simulink model "AR4_robotv5"  (R2021a)
settings: Solver=VariableStepAuto  StartTime=0.0  StopTime=13.7896  RelTol=1e-3
undefined symbols (not defined in the file or in its folder): B, Levenberg, Marquardt, sigbuilder_block, Spline, X, Y, Z
libraries: sm_lib x612, nesl_utility x123, robotcorelib x28, simulink_extras x19, simulink x17, robotmaniplib x9
(part 13 of 14)

== system AR4_robotv5/Subsystem8/link4 ==
  Inertia : sm_lib/Body Elements/Inertia  InertiaType=Custom  Mass=0.330915774998875  MassUnits=kg  CenterOfMass=[0, 0, 0]  CenterOfMassUnits=m  MomentsOfInertia=[0.0007707144648363029, 0.000143595801102121, 0.00078144566914053]  MomentsOfInertiaUnits=kg*m^2  ProductsOfInertia=[6.92144604392256e-05, -9.03681380466358e-09, -5.83780279549621e-08]  ProductsOfInertiaUnits=kg*m^2  GraphicType=None  MarkerShape=Inertia  MarkerSize=20  GraphicVisPropType=SimpleVisualProperties  GraphicDiffuseColor=[0.5 0.5 0.5]  GraphicSpecularColor=[0.5 0.5 0.5 1.0]  GraphicAmbientColor=[0.15 0.15 0.15 1.0]  GraphicEmissiveColor=[0.0 0.0 0.0 1.0]  GraphicShininess=75  GraphicOpacity=1.0
  InertiaOriginTransform : sm_lib/Frames and Transforms/Rigid Transform  TranslationMethod=Cartesian  TranslationStandardOffset=0  TranslationLengthUnit=m  TranslationStandardAxis=+Z  TranslationCartesianOffset=[1.65972746341003e-06, 0.114308868744708, -0.00196391551724488]  TranslationROffset=0  TranslationROffsetUnits=m  TranslationZOffset=0  TranslationZOffsetUnits=m  TranslationThetaOffset=0  TranslationThetaOffsetUnits=deg  RotationMethod=RotationSequence  RotationAngleUnits=deg  RotationStandardAxis=+Z  RotationAngle=0.0  RotationArbitraryAxis=[0 0 1]  FollAlignAxisA=+X  BaseAlignAxisA=+Y  FollAlignAxisB=+Y  BaseAlignAxisB=+Z  RotationSequenceAxes=BaseAxes  RotationSequence=XYZ  RotationSequenceAngles=[0, 0, 0]  RotationSequenceAnglesUnits=rad  RotationMatrix=[1 0 0; 0 1 0; 0 0 1]
  ReferenceFrame : sm_lib/Frames and Transforms/Reference Frame
  Visual : sm_lib/Body Elements/File Solid  ExtGeomFileName=AR4_robotv5/meshes/link4.STL  UnitType=Custom  ExtGeomFileUnits=m  StepReaderType=HEX  ExportConvexHullGeometry=off  InertiaType=Custom  Mass=0  MassUnits=kg  CenterOfMass=[0, 0, 0]  CenterOfMassUnits=m  MomentsOfInertia=[0, 0, 0]  MomentsOfInertiaUnits=kg*m^2  ProductsOfInertia=[0, 0, 0]  ProductsOfInertiaUnits=kg*m^2  BasedOnType=DensityFromFile  Density=1000  DensityUnits=kg/m^3  DoExposeReferenceFrame=on  SerializedFrames=<Frames/>  GraphicType=FromGeometry  MarkerShape=Sphere  MarkerSize=10  GraphicVisPropType=SimpleVisualProperties  GraphicDiffuseColor=[0.792156862745098, 0.819607843137255, 0.933333333333333]  GraphicSpecularColor=[0.5 0.5 0.5 1.0]  GraphicAmbientColor=[0.15 0.15 0.15 1.0]  GraphicEmissiveColor=[0.0 0.0 0.0 1.0]  GraphicShininess=75  GraphicOpacity=1
  VisualOriginTransform : sm_lib/Frames and Transforms/Rigid Transform  TranslationMethod=Cartesian  TranslationStandardOffset=0  TranslationLengthUnit=m  TranslationStandardAxis=+Z  TranslationCartesianOffset=[0, 0, 0]  TranslationROffset=0  TranslationROffsetUnits=m  TranslationZOffset=0  TranslationZOffsetUnits=m  TranslationThetaOffset=0  TranslationThetaOffsetUnits=deg  RotationMethod=RotationSequence  RotationAngleUnits=deg  RotationStandardAxis=+Z  RotationAngle=0.0  RotationArbitraryAxis=[0 0 1]  FollAlignAxisA=+X  BaseAlignAxisA=+Y  FollAlignAxisB=+Y  BaseAlignAxisB=+Z  RotationSequenceAxes=BaseAxes  RotationSequence=XYZ  RotationSequenceAngles=[0, 0, 0]  RotationSequenceAnglesUnits=rad  RotationMatrix=[1 0 0; 0 1 0; 0 0 1]
  j4_AxisInvTransform : sm_lib/Frames and Transforms/Rigid Transform  TranslationMethod=Cartesian  TranslationStandardOffset=0  TranslationLengthUnit=m  TranslationStandardAxis=+Z  TranslationCartesianOffset=[0, 0, 0]  TranslationROffset=0  TranslationROffsetUnits=m  TranslationZOffset=0  TranslationZOffsetUnits=m  TranslationThetaOffset=0  TranslationThetaOffsetUnits=deg  RotationMethod=ArbitraryAxis  RotationAngleUnits=rad  RotationStandardAxis=+Z  RotationAngle=1.570796326794897  RotationArbitraryAxis=[-1, 0, 0]  FollAlignAxisA=+X  BaseAlignAxisA=+Y  FollAlignAxisB=+Y  BaseAlignAxisB=+Z  RotationSequenceAxes=FollowerAxes  RotationSequence=XYX  RotationSequenceAngles=[0 0 0]  RotationSequenceAnglesUnits=deg  RotationMatrix=[1 0 0; 0 1 0; 0 0 1]
  j5_AxisTransform : sm_lib/Frames and Transforms/Rigid Transform  TranslationMethod=Cartesian  TranslationStandardOffset=0  TranslationLengthUnit=m  TranslationStandardAxis=+Z  TranslationCartesianOffset=[0, 0, 0]  TranslationROffset=0  TranslationROffsetUnits=m  TranslationZOffset=0  TranslationZOffsetUnits=m  TranslationThetaOffset=0  TranslationThetaOffsetUnits=deg  RotationMethod=ArbitraryAxis  RotationAngleUnits=rad  RotationStandardAxis=+Z  RotationAngle=1.570796326794897  RotationArbitraryAxis=[-1, 0, 0]  FollAlignAxisA=+X  BaseAlignAxisA=+Y  FollAlignAxisB=+Y  BaseAlignAxisB=+Z  RotationSequenceAxes=FollowerAxes  RotationSequence=XYX  RotationSequenceAngles=[0 0 0]  RotationSequenceAnglesUnits=deg  RotationMatrix=[1 0 0; 0 1 0; 0 0 1]
  j5_OriginTransform : sm_lib/Frames and Transforms/Rigid Transform  TranslationMethod=Cartesian  TranslationStandardOffset=0  TranslationLengthUnit=m  TranslationStandardAxis=+Z  TranslationCartesianOffset=[0, 0.225041312909753, 0.0007499997333115]  TranslationROffset=0  TranslationROffsetUnits=m  TranslationZOffset=0  TranslationZOffsetUnits=m  TranslationThetaOffset=0  TranslationThetaOffsetUnits=deg  RotationMethod=RotationSequence  RotationAngleUnits=deg  RotationStandardAxis=+Z  RotationAngle=0.0  RotationArbitraryAxis=[0 0 1]  FollAlignAxisA=+X  BaseAlignAxisA=+Y  FollAlignAxisB=+Y  BaseAlignAxisB=+Z  RotationSequenceAxes=BaseAxes  RotationSequence=XYZ  RotationSequenceAngles=[1.57079631189374, -0.000843332253807779, 0]  RotationSequenceAnglesUnits=rad  RotationMatrix=[1 0 0; 0 1 0; 0 0 1]
  F : PMIOPort  Side=Left
  F1 : PMIOPort  Port=2  Side=Right
  connections:
  j5_AxisTransform/LConn1 -- j5_OriginTransform/RConn1
  j5_AxisTransform/RConn1 -- F1/RConn1
  j4_AxisInvTransform/RConn1 -- F/RConn1
  Visual/RConn1 -- VisualOriginTransform/RConn1
  j5_OriginTransform/LConn1 -- j4_AxisInvTransform/LConn1 -- VisualOriginTransform/LConn1 -- ReferenceFrame/RConn1 -- InertiaOriginTransform/LConn1
  Inertia/RConn1 -- InertiaOriginTransform/RConn1

== system AR4_robotv5/Subsystem8/link5 ==
  Inertia : sm_lib/Body Elements/Inertia  InertiaType=Custom  Mass=0.0245034490928621  MassUnits=kg  CenterOfMass=[0, 0, 0]  CenterOfMassUnits=m  MomentsOfInertia=[9.036336684299629e-06, 5.7526255063883e-06, 1.2157538793257e-05]  MomentsOfInertiaUnits=kg*m^2  ProductsOfInertia=[-2.03350961333318e-08, -2.14953206266449e-09, 9.04257798543254e-09]  ProductsOfInertiaUnits=kg*m^2  GraphicType=None  MarkerShape=Inertia  MarkerSize=20  GraphicVisPropType=SimpleVisualProperties  GraphicDiffuseColor=[0.5 0.5 0.5]  GraphicSpecularColor=[0.5 0.5 0.5 1.0]  GraphicAmbientColor=[0.15 0.15 0.15 1.0]  GraphicEmissiveColor=[0.0 0.0 0.0 1.0]  GraphicShininess=75  GraphicOpacity=1.0
  InertiaOriginTransform : sm_lib/Frames and Transforms/Rigid Transform  TranslationMethod=Cartesian  TranslationStandardOffset=0  TranslationLengthUnit=m  TranslationStandardAxis=+Z  TranslationCartesianOffset=[4.46631409203313e-05, 0.0010582355958296, -0.000637441503684444]  TranslationROffset=0  TranslationROffsetUnits=m  TranslationZOffset=0  TranslationZOffsetUnits=m  TranslationThetaOffset=0  TranslationThetaOffsetUnits=deg  RotationMethod=RotationSequence  RotationAngleUnits=deg  RotationStandardAxis=+Z  RotationAngle=0.0  RotationArbitraryAxis=[0 0 1]  FollAlignAxisA=+X  BaseAlignAxisA=+Y  FollAlignAxisB=+Y  BaseAlignAxisB=+Z  RotationSequenceAxes=BaseAxes  RotationSequence=XYZ  RotationSequenceAngles=[0, 0, 0]  RotationSequenceAnglesUnits=rad  RotationMatrix=[1 0 0; 0 1 0; 0 0 1]
  ReferenceFrame : sm_lib/Frames and Transforms/Reference Frame
  Visual : sm_lib/Body Elements/File Solid  ExtGeomFileName=AR4_robotv5/meshes/link5.STL  UnitType=Custom  ExtGeomFileUnits=m  StepReaderType=HEX  ExportConvexHullGeometry=off  InertiaType=Custom  Mass=0  MassUnits=kg  CenterOfMass=[0, 0, 0]  CenterOfMassUnits=m  MomentsOfInertia=[0, 0, 0]  MomentsOfInertiaUnits=kg*m^2  ProductsOfInertia=[0, 0, 0]  ProductsOfInertiaUnits=kg*m^2  BasedOnType=DensityFromFile  Density=1000  DensityUnits=kg/m^3  DoExposeReferenceFrame=on  SerializedFrames=<Frames/>  GraphicType=FromGeometry  MarkerShape=Sphere  MarkerSize=10  GraphicVisPropType=SimpleVisualProperties  GraphicDiffuseColor=[0.792156862745098, 0.819607843137255, 0.933333333333333]  GraphicSpecularColor=[0.5 0.5 0.5 1.0]  GraphicAmbientColor=[0.15 0.15 0.15 1.0]  GraphicEmissiveColor=[0.0 0.0 0.0 1.0]  GraphicShininess=75  GraphicOpacity=1
  VisualOriginTransform : sm_lib/Frames and Transforms/Rigid Transform  TranslationMethod=Cartesian  TranslationStandardOffset=0  TranslationLengthUnit=m  TranslationStandardAxis=+Z  TranslationCartesianOffset=[0, 0, 0]  TranslationROffset=0  TranslationROffsetUnits=m  TranslationZOffset=0  TranslationZOffsetUnits=m  TranslationThetaOffset=0  TranslationThetaOffsetUnits=deg  RotationMethod=RotationSequence  RotationAngleUnits=deg  RotationStandardAxis=+Z  RotationAngle=0.0  RotationArbitraryAxis=[0 0 1]  FollAlignAxisA=+X  BaseAlignAxisA=+Y  FollAlignAxisB=+Y  BaseAlignAxisB=+Z  RotationSequenceAxes=BaseAxes  RotationSequence=XYZ  RotationSequenceAngles=[0, 0, 0]  RotationSequenceAnglesUnits=rad  RotationMatrix=[1 0 0; 0 1 0; 0 0 1]
  j5_AxisInvTransform : sm_lib/Frames and Transforms/Rigid Transform  TranslationMethod=Cartesian  TranslationStandardOffset=0  TranslationLengthUnit=m  TranslationStandardAxis=+Z  TranslationCartesianOffset=[0, 0, 0]  TranslationROffset=0  TranslationROffsetUnits=m  TranslationZOffset=0  TranslationZOffsetUnits=m  TranslationThetaOffset=0  TranslationThetaOffsetUnits=deg  RotationMethod=ArbitraryAxis  RotationAngleUnits=rad  RotationStandardAxis=+Z  RotationAngle=1.570796326794897  RotationArbitraryAxis=[-1, 0, 0]  FollAlignAxisA=+X  BaseAlignAxisA=+Y  FollAlignAxisB=+Y  BaseAlignAxisB=+Z  RotationSequenceAxes=FollowerAxes  RotationSequence=XYX  RotationSequenceAngles=[0 0 0]  RotationSequenceAnglesUnits=deg  RotationMatrix=[1 0 0; 0 1 0; 0 0 1]
  j6_AxisTransform : sm_lib/Frames and Transforms/Rigid Transform  TranslationMethod=Cartesian  TranslationStandardOffset=0  TranslationLengthUnit=m  TranslationStandardAxis=+Z  TranslationCartesianOffset=[0, 0, 0]  TranslationROffset=0  TranslationROffsetUnits=m  TranslationZOffset=0  TranslationZOffsetUnits=m  TranslationThetaOffset=0  TranslationThetaOffsetUnits=deg  RotationMethod=ArbitraryAxis  RotationAngleUnits=rad  RotationStandardAxis=+Z  RotationAngle=0  RotationArbitraryAxis=[1, 0, 0]  FollAlignAxisA=+X  BaseAlignAxisA=+Y  FollAlignAxisB=+Y  BaseAlignAxisB=+Z  RotationSequenceAxes=FollowerAxes  RotationSequence=XYX  RotationSequenceAngles=[0 0 0]  RotationSequenceAnglesUnits=deg  RotationMatrix=[1 0 0; 0 1 0; 0 0 1]
  j6_OriginTransform : sm_lib/Frames and Transforms/Rigid Transform  TranslationMethod=Cartesian  TranslationStandardOffset=0  TranslationLengthUnit=m  TranslationStandardAxis=+Z  TranslationCartesianOffset=[0, 0, 0]  TranslationROffset=0  TranslationROffsetUnits=m  TranslationZOffset=0  TranslationZOffsetUnits=m  TranslationThetaOffset=0  TranslationThetaOffsetUnits=deg  RotationMethod=RotationSequence  RotationAngleUnits=deg  RotationStandardAxis=+Z  RotationAngle=0.0  RotationArbitraryAxis=[0 0 1]  FollAlignAxisA=+X  BaseAlignAxisA=+Y  FollAlignAxisB=+Y  BaseAlignAxisB=+Z  RotationSequenceAxes=BaseAxes  RotationSequence=XYZ  RotationSequenceAngles=[0, 0, 3.14159265358979]  RotationSequenceAnglesUnits=rad  RotationMatrix=[1 0 0; 0 1 0; 0 0 1]
  F : PMIOPort  Side=Left
  F1 : PMIOPort  Port=2  Side=Right
  connections:
  j6_AxisTransform/LConn1 -- j6_OriginTransform/RConn1
  j6_AxisTransform/RConn1 -- F1/RConn1
  j5_AxisInvTransform/RConn1 -- F/RConn1
  Visual/RConn1 -- VisualOriginTransform/RConn1
  j6_OriginTransform/LConn1 -- j5_AxisInvTransform/LConn1 -- VisualOriginTransform/LConn1 -- ReferenceFrame/RConn1 -- InertiaOriginTransform/LConn1
  Inertia/RConn1 -- InertiaOriginTransform/RConn1

== system AR4_robotv5/Subsystem8/link6 ==
  Inertia : sm_lib/Body Elements/Inertia  InertiaType=Custom  Mass=0.121376042767568  MassUnits=kg  CenterOfMass=[0, 0, 0]  CenterOfMassUnits=m  MomentsOfInertia=[3.53039178237827e-05, 1.81330403322111e-05, 4.26315107565952e-05]  MomentsOfInertiaUnits=kg*m^2  ProductsOfInertia=[-2.21518225549172e-07, -4.47726039625278e-07, -4.7308746638171e-08]  ProductsOfInertiaUnits=kg*m^2  GraphicType=None  MarkerShape=Inertia  MarkerSize=20  GraphicVisPropType=SimpleVisualProperties  GraphicDiffuseColor=[0.5 0.5 0.5]  GraphicSpecularColor=[0.5 0.5 0.5 1.0]  GraphicAmbientColor=[0.15 0.15 0.15 1.0]  GraphicEmissiveColor=[0.0 0.0 0.0 1.0]  GraphicShininess=75  GraphicOpacity=1.0
  InertiaOriginTransform : sm_lib/Frames and Transforms/Rigid Transform  TranslationMethod=Cartesian  TranslationStandardOffset=0  TranslationLengthUnit=m  TranslationStandardAxis=+Z  TranslationCartesianOffset=[-0.00160633858276565, -0.000457062617008543, -0.0587695487539506]  TranslationROffset=0  TranslationROffsetUnits=m  TranslationZOffset=0  TranslationZOffsetUnits=m  TranslationThetaOffset=0  TranslationThetaOffsetUnits=deg  RotationMethod=RotationSequence  RotationAngleUnits=deg  RotationStandardAxis=+Z  RotationAngle=0.0  RotationArbitraryAxis=[0 0 1]  FollAlignAxisA=+X  BaseAlignAxisA=+Y  FollAlignAxisB=+Y  BaseAlignAxisB=+Z  RotationSequenceAxes=BaseAxes  RotationSequence=XYZ  RotationSequenceAngles=[0, 0, 0]  RotationSequenceAnglesUnits=rad  RotationMatrix=[1 0 0; 0 1 0; 0 0 1]
  ReferenceFrame : sm_lib/Frames and Transforms/Reference Frame
  Visual : sm_lib/Body Elements/File Solid  ExtGeomFileName=AR4_robotv5/meshes/link6.STL  UnitType=Custom  ExtGeomFileUnits=m  StepReaderType=HEX  ExportConvexHullGeometry=off  InertiaType=Custom  Mass=0  MassUnits=kg  CenterOfMass=[0, 0, 0]  CenterOfMassUnits=m  MomentsOfInertia=[0, 0, 0]  MomentsOfInertiaUnits=kg*m^2  ProductsOfInertia=[0, 0, 0]  ProductsOfInertiaUnits=kg*m^2  BasedOnType=DensityFromFile  Density=1000  DensityUnits=kg/m^3  DoExposeReferenceFrame=on  SerializedFrames=<Frames/>  GraphicType=FromGeometry  MarkerShape=Sphere  MarkerSize=10  GraphicVisPropType=SimpleVisualProperties  GraphicDiffuseColor=[0.792156862745098, 0.819607843137255, 0.933333333333333]  GraphicSpecularColor=[0.5 0.5 0.5 1.0]  GraphicAmbientColor=[0.15 0.15 0.15 1.0]  GraphicEmissiveColor=[0.0 0.0 0.0 1.0]  GraphicShininess=75  GraphicOpacity=1
  VisualOriginTransform : sm_lib/Frames and Transforms/Rigid Transform  TranslationMethod=Cartesian  TranslationStandardOffset=0  TranslationLengthUnit=m  TranslationStandardAxis=+Z  TranslationCartesianOffset=[0, 0, 0]  TranslationROffset=0  TranslationROffsetUnits=m  TranslationZOffset=0  TranslationZOffsetUnits=m  TranslationThetaOffset=0  TranslationThetaOffsetUnits=deg  RotationMethod=RotationSequence  RotationAngleUnits=deg  RotationStandardAxis=+Z  RotationAngle=0.0  RotationArbitraryAxis=[0 0 1]  FollAlignAxisA=+X  BaseAlignAxisA=+Y  FollAlignAxisB=+Y  BaseAlignAxisB=+Z  RotationSequenceAxes=BaseAxes  RotationSequence=XYZ  RotationSequenceAngles=[0, 0, 0]  RotationSequenceAnglesUnits=rad  RotationMatrix=[1 0 0; 0 1 0; 0 0 1]
  j6_AxisInvTransform : sm_lib/Frames and Transforms/Rigid Transform  TranslationMethod=Cartesian  TranslationStandardOffset=0  TranslationLengthUnit=m  TranslationStandardAxis=+Z  TranslationCartesianOffset=[0, 0, 0]  TranslationROffset=0  TranslationROffsetUnits=m  TranslationZOffset=0  TranslationZOffsetUnits=m  TranslationThetaOffset=0  TranslationThetaOffsetUnits=deg  RotationMethod=ArbitraryAxis  RotationAngleUnits=rad  RotationStandardAxis=+Z  RotationAngle=0  RotationArbitraryAxis=[1, 0, 0]  FollAlignAxisA=+X  BaseAlignAxisA=+Y  FollAlignAxisB=+Y  BaseAlignAxisB=+Z  RotationSequenceAxes=FollowerAxes  RotationSequence=XYX  RotationSequenceAngles=[0 0 0]  RotationSequenceAnglesUnits=deg  RotationMatrix=[1 0 0; 0 1 0; 0 0 1]
  j7_OriginTransform : sm_lib/Frames and Transforms/Rigid Transform  TranslationMethod=Cartesian  TranslationStandardOffset=0  TranslationLengthUnit=m  TranslationStandardAxis=+Z  TranslationCartesianOffset=[0, -0.000201201957805657, -0.0848321039170631]  TranslationROffset=0  TranslationROffsetUnits=m  TranslationZOffset=0  TranslationZOffsetUnits=m  TranslationThetaOffset=0  TranslationThetaOffsetUnits=deg  RotationMethod=RotationSequence  RotationAngleUnits=deg  RotationStandardAxis=+Z  RotationAngle=0.0  RotationArbitraryAxis=[0 0 1]  FollAlignAxisA=+X  BaseAlignAxisA=+Y  FollAlignAxisB=+Y  BaseAlignAxisB=+Z  RotationSequenceAxes=BaseAxes  RotationSequence=XYZ  RotationSequenceAngles=[0, 1.5707963267949, 0]  RotationSequenceAnglesUnits=rad  RotationMatrix=[1 0 0; 0 1 0; 0 0 1]
  F : PMIOPort  Side=Left
  F1 : PMIOPort  Port=2  Side=Right
  connections:
  j7_OriginTransform/RConn1 -- F1/RConn1
  j6_AxisInvTransform/RConn1 -- F/RConn1
  Visual/RConn1 -- VisualOriginTransform/RConn1
  j7_OriginTransform/LConn1 -- j6_AxisInvTransform/LConn1 -- VisualOriginTransform/LConn1 -- ReferenceFrame/RConn1 -- InertiaOriginTransform/LConn1
  Inertia/RConn1 -- InertiaOriginTransform/RConn1

== system AR4_robotv5/Subsystem8/link7 ==
  Inertia : sm_lib/Body Elements/Inertia  InertiaType=Custom  Mass=4.28541445828409e-05  MassUnits=kg  CenterOfMass=[0, 0, 0]  CenterOfMassUnits=m  MomentsOfInertia=[3.26374304335892e-11, 3.40574299802589e-10, 3.40574299802589e-10]  MomentsOfInertiaUnits=kg*m^2  ProductsOfInertia=[2.22599419002211e-28, 4.70953291237086e-24, 1.38439272082023e-24]  ProductsOfInertiaUnits=kg*m^2  GraphicType=None  MarkerShape=Inertia  MarkerSize=20  GraphicVisPropType=SimpleVisualProperties  GraphicDiffuseColor=[0.5 0.5 0.5]  GraphicSpecularColor=[0.5 0.5 0.5 1.0]  GraphicAmbientColor=[0.15 0.15 0.15 1.0]  GraphicEmissiveColor=[0.0 0.0 0.0 1.0]  GraphicShininess=75  GraphicOpacity=1.0
  InertiaOriginTransform : sm_lib/Frames and Transforms/Rigid Transform  TranslationMethod=Cartesian  TranslationStandardOffset=0  TranslationLengthUnit=m  TranslationStandardAxis=+Z  TranslationCartesianOffset=[0.00401715386268953, -1.82145964977565e-17, -1.11022302462516e-16]  TranslationROffset=0  TranslationROffsetUnits=m  TranslationZOffset=0  TranslationZOffsetUnits=m  TranslationThetaOffset=0  TranslationThetaOffsetUnits=deg  RotationMethod=RotationSequence  RotationAngleUnits=deg  RotationStandardAxis=+Z  RotationAngle=0.0  RotationArbitraryAxis=[0 0 1]  FollAlignAxisA=+X  BaseAlignAxisA=+Y  FollAlignAxisB=+Y  BaseAlignAxisB=+Z  RotationSequenceAxes=BaseAxes  RotationSequence=XYZ  RotationSequenceAngles=[0, 0, 0]  RotationSequenceAnglesUnits=rad  RotationMatrix=[1 0 0; 0 1 0; 0 0 1]
  ReferenceFrame : sm_lib/Frames and Transforms/Reference Frame
  Visual : sm_lib/Body Elements/File Solid  ExtGeomFileName=AR4_robotv5/meshes/link7.STL  UnitType=Custom  ExtGeomFileUnits=m  StepReaderType=HEX  ExportConvexHullGeometry=off  InertiaType=Custom  Mass=0  MassUnits=kg  CenterOfMass=[0, 0, 0]  CenterOfMassUnits=m  MomentsOfInertia=[0, 0, 0]  MomentsOfInertiaUnits=kg*m^2  ProductsOfInertia=[0, 0, 0]  ProductsOfInertiaUnits=kg*m^2  BasedOnType=DensityFromFile  Density=1000  DensityUnits=kg/m^3  DoExposeReferenceFrame=on  SerializedFrames=<Frames/>  GraphicType=FromGeometry  MarkerShape=Sphere  MarkerSize=10  GraphicVisPropType=SimpleVisualProperties  GraphicDiffuseColor=[0.792156862745098, 0.819607843137255, 0.933333333333333]  GraphicSpecularColor=[0.5 0.5 0.5 1.0]  GraphicAmbientColor=[0.15 0.15 0.15 1.0]  GraphicEmissiveColor=[0.0 0.0 0.0 1.0]  GraphicShininess=75  GraphicOpacity=1
  VisualOriginTransform : sm_lib/Frames and Transforms/Rigid Transform  TranslationMethod=Cartesian  TranslationStandardOffset=0  TranslationLengthUnit=m  TranslationStandardAxis=+Z  TranslationCartesianOffset=[0, 0, 0]  TranslationROffset=0  TranslationROffsetUnits=m  TranslationZOffset=0  TranslationZOffsetUnits=m  TranslationThetaOffset=0  TranslationThetaOffsetUnits=deg  RotationMethod=RotationSequence  RotationAngleUnits=deg  RotationStandardAxis=+Z  RotationAngle=0.0  RotationArbitraryAxis=[0 0 1]  FollAlignAxisA=+X  BaseAlignAxisA=+Y  FollAlignAxisB=+Y  BaseAlignAxisB=+Z  RotationSequenceAxes=BaseAxes  RotationSequence=XYZ  RotationSequenceAngles=[0, 0, 0]  RotationSequenceAnglesUnits=rad  RotationMatrix=[1 0 0; 0 1 0; 0 0 1]
  F : PMIOPort  Side=Left
  connections:
  Visual/RConn1 -- VisualOriginTransform/RConn1
  F/RConn1 -- VisualOriginTransform/LConn1 -- ReferenceFrame/RConn1 -- InertiaOriginTransform/LConn1
  Inertia/RConn1 -- InertiaOriginTransform/RConn1

== matlab function AR4_robotv5/Subsystem6/MATLAB Function4 ==
  data: theta1 input; H output; theta2 input; theta3 input; theta4 input; theta5 input; theta6 input; X output; Y output; Z output; Rz output; Ry output; Rx output
function [H, X, Y, Z, Rz, Ry, Rx] = forward_kinematics_AR4(theta1, theta2, theta3, theta4, theta5, theta6)
% forward_kinematics_AR4 Computes the forward kinematics for the AR4 robot.
%
%   [H, X, Y, Z, Rz, Ry, Rx] = forward_kinematics_AR4(theta1, theta2, theta3, theta4, theta5, theta6)
%
%   Inputs:
%       theta1, theta2, theta3, theta4, theta5, theta6 - Joint angles (degrees)
%
%   Outputs:
%       H  - 4x4 homogeneous transformation matrix of the end-effector (mm)
%       X, Y, Z - End-effector position coordinates (mm)
%       Rz, Ry, Rx - End-effector orientation angles in degrees (ZYX Euler angles)
%
%   The AR4 robot parameters (in mm) used here are:
%       a1 = 64.2;   a2 = 305;    a3 = 0;
%       d1 = 151.27; d4 = 225.04; d6 = 37.9;
%
%   The DH parameters are defined as:
%       Joint 1: [theta1,         d1, a1, -90]
%       Joint 2: [theta2 - 90,     0,  a2,   0]
%       Joint 3: [theta3 + 180,    0,  a3,  90]
%       Joint 4: [theta4,         d4,  0,   -90]
%       Joint 5: [theta5,          0,  0,    90]
%       Joint 6: [theta6,         d6,  0,     0]

    %% Robot parameters
    a1 = 64.2;     a2 = 305;    a3 = 0;
    d1 = 151.27;   d4 = 225.04; d6 = 84.832;

    %% DH parameters
    DH1 = [theta1,       d1, a1, -90];
    DH2 = [theta2 - 90,  0,  a2,   0];
    DH3 = [theta3 + 180, 0,  a3,  90];
    DH4 = [theta4,       d4,  0,   -90];
    DH5 = [theta5,        0,  0,    90];
    DH6 = [theta6,       d6,  0,     0];

    %% Compute transformations
    A1 = computeDH(DH1);
    A2 = computeDH(DH2);
    A3 = computeDH(DH3);
    A4 = computeDH(DH4);
    A5 = computeDH(DH5);
    A6 = computeDH(DH6);

    H = A1 * A2 * A3 * A4 * A5 * A6;

    %% Extract position
    X = H(1,4);
    Y = H(2,4);
    Z = H(3,4);

    %% Extract orientation (ZYX Euler angles in degrees)
    R = H(1:3, 1:3);
    
    % Calculate Ry (pitch)
    Ry = atan2d(-R(3,1), sqrt(R(3,2)^2 + R(3,3)^2));
    
    % Check for gimbal lock (pitch near ±90°)
    if abs(abs(Ry) - 90) < eps
        % Gimbal lock case - set yaw to 0 and compute roll from alternate terms
        Rz = 0;
        Rx = atan2d(R(1,2), R(2,2));
    else
        % Normal case
        Rz = atan2d(R(2,1), R(1,1));
        Rx = atan2d(R(3,2), R(3,3));
    end
end

function A = computeDH(dh)
    theta = dh(1);
    d     = dh(2);
    a     = dh(3);
    alpha = dh(4);
    
    A = [cosd(theta), -sind(theta)*cosd(alpha),  sind(theta)*sind(alpha), a*cosd(theta);
         sind(theta),  cosd(theta)*cosd(alpha), -cosd(theta)*sind(alpha), a*sind(theta);
         0,            sind(alpha),             cosd(alpha),             d;
         0,            0,                       0,                       1];
end

== matlab function AR4_robotv5/MATLAB Function3 ==
  data: theta1 input; H output; theta2 input; theta3 input; theta4 input; theta5 input; theta6 input; X output; Y output; Z output; Rz output; Ry output; Rx output
function [H, X, Y, Z, Rz, Ry, Rx] = forward_kinematics_AR4(theta1, theta2, theta3, theta4, theta5, theta6)
% forward_kinematics_AR4 Computes the forward kinematics for the AR4 robot.
%
%   [H, X, Y, Z, Rz, Ry, Rx] = forward_kinematics_AR4(theta1, theta2, theta3, theta4, theta5, theta6)
%
%   Inputs:
%       theta1, theta2, theta3, theta4, theta5, theta6 - Joint angles (degrees)
%
%   Outputs:
%       H  - 4x4 homogeneous transformation matrix of the end-effector (mm)
%       X, Y, Z - End-effector position coordinates (mm)
%       Rz, Ry, Rx - End-effector orientation angles in degrees (ZYX Euler angles)
%
%   The AR4 robot parameters (in mm) used here are:
%       a1 = 64.2;   a2 = 305;    a3 = 0;
%       d1 = 151.27; d4 = 225.04; d6 = 37.9;
%
%   The DH parameters are defined as:
%       Joint 1: [theta1,         d1, a1, -90]
%       Joint 2: [theta2 - 90,     0,  a2,   0]
%       Joint 3: [theta3 + 180,    0,  a3,  90]
%       Joint 4: [theta4,         d4,  0,   -90]
%       Joint 5: [theta5,          0,  0,    90]
%       Joint 6: [theta6,         d6,  0,     0]

    %% Robot parameters
    a1 = 64.2;     a2 = 305;    a3 = 0;
    d1 = 151.27;   d4 = 225.04; d6 = 84.832;

    %% DH parameters
    DH1 = [theta1,       d1, a1, -90];
    DH2 = [theta2 - 90,  0,  a2,   0];
    DH3 = [theta3 + 180, 0,  a3,  90];
    DH4 = [theta4,       d4,  0,   -90];
    DH5 = [theta5,        0,  0,    90];
    DH6 = [theta6,       d6,  0,     0];

    %% Compute transformations
    A1 = computeDH(DH1);
    A2 = computeDH(DH2);
    A3 = computeDH(DH3);
    A4 = computeDH(DH4);
    A5 = computeDH(DH5);
    A6 = computeDH(DH6);

    H = A1 * A2 * A3 * A4 * A5 * A6;

    %% Extract position
    X = H(1,4);
    Y = H(2,4);
    Z = H(3,4);

    %% Extract orientation (ZYX Euler angles in degrees)
    R = H(1:3, 1:3);
    
    % Calculate Ry (pitch)
    Ry = atan2d(-R(3,1), sqrt(R(3,2)^2 + R(3,3)^2));
    
    % Check for gimbal lock (pitch near ±90°)
    if abs(abs(Ry) - 90) < eps
        % Gimbal lock case - set yaw to 0 and compute roll from alternate terms
        Rz = 0;
        Rx = atan2d(R(1,2), R(2,2));
    else
        % Normal case
        Rz = atan2d(R(2,1), R(1,1));
        Rx = atan2d(R(3,2), R(3,3));
    end
end

function A = computeDH(dh)
    theta = dh(1);
    d     = dh(2);
    a     = dh(3);
    alpha = dh(4);
    
    A = [cosd(theta), -sind(theta)*cosd(alpha),  sind(theta)*sind(alpha), a*cosd(theta);
         sind(theta),  cosd(theta)*cosd(alpha), -cosd(theta)*sind(alpha), a*sind(theta);
         0,            sind(alpha),             cosd(alpha),             d;
         0,            0,                       0,                       1];
end

== matlab function AR4_robotv5/MATLAB Function6 ==
  data: theta1 input; H output; theta2 input; theta3 input; theta4 input; theta5 input; theta6 input; X output; Y output; Z output; Rz output; Ry output; Rx output
function [H, X, Y, Z, Rz, Ry, Rx] = forward_kinematics_AR4(theta1, theta2, theta3, theta4, theta5, theta6)
% forward_kinematics_AR4 Computes the forward kinematics for the AR4 robot.
%
%   [H, X, Y, Z, Rz, Ry, Rx] = forward_kinematics_AR4(theta1, theta2, theta3, theta4, theta5, theta6)
%
%   Inputs:
%       theta1, theta2, theta3, theta4, theta5, theta6 - Joint angles (degrees)
%
%   Outputs:
%       H  - 4x4 homogeneous transformation matrix of the end-effector (mm)
%       X, Y, Z - End-effector position coordinates (mm)
%       Rz, Ry, Rx - End-effector orientation angles in degrees (ZYX Euler angles)
%
%   The AR4 robot parameters (in mm) used here are:
%       a1 = 64.2;   a2 = 305;    a3 = 0;
%       d1 = 151.27; d4 = 225.04; d6 = 37.9;
%
%   The DH parameters are defined as:
%       Joint 1: [theta1,         d1, a1, -90]
%       Joint 2: [theta2 - 90,     0,  a2,   0]
%       Joint 3: [theta3 + 180,    0,  a3,  90]
%       Joint 4: [theta4,         d4,  0,   -90]
%       Joint 5: [theta5,          0,  0,    90]
%       Joint 6: [theta6,         d6,  0,     0]

    %% Robot parameters
    a1 = 64.2;     a2 = 305;    a3 = 0;
    d1 = 151.27;   d4 = 225.04; d6 = 84.832;

    %% DH parameters
    DH1 = [theta1,       d1, a1, -90];
    DH2 = [theta2 - 90,  0,  a2,   0];
    DH3 = [theta3 + 180, 0,  a3,  90];
    DH4 = [theta4,       d4,  0,   -90];
    DH5 = [theta5,        0,  0,    90];
    DH6 = [theta6,       d6,  0,     0];

    %% Compute transformations
    A1 = computeDH(DH1);
    A2 = computeDH(DH2);
    A3 = computeDH(DH3);
    A4 = computeDH(DH4);
    A5 = computeDH(DH5);
    A6 = computeDH(DH6);

    H = A1 * A2 * A3 * A4 * A5 * A6;

    %% Extract position
    X = H(1,4);
    Y = H(2,4);
    Z = H(3,4);

    %% Extract orientation (ZYX Euler angles in degrees)
    R = H(1:3, 1:3);
    
    % Calculate Ry (pitch)
    Ry = atan2d(-R(3,1), sqrt(R(3,2)^2 + R(3,3)^2));
    
    % Check for gimbal lock (pitch near ±90°)
    if abs(abs(Ry) - 90) < eps
        % Gimbal lock case - set yaw to 0 and compute roll from alternate terms
        Rz = 0;
        Rx = atan2d(R(1,2), R(2,2));
    else
        % Normal case
        Rz = atan2d(R(2,1), R(1,1));
        Rx = atan2d(R(3,2), R(3,3));
    end
end

function A = computeDH(dh)
    theta = dh(1);
    d     = dh(2);
    a     = dh(3);
    alpha = dh(4);
    
    A = [cosd(theta), -sind(theta)*cosd(alpha),  sind(theta)*sind(alpha), a*cosd(theta);
         sind(theta),  cosd(theta)*cosd(alpha), -cosd(theta)*sind(alpha), a*sind(theta);
         0,            sind(alpha),             cosd(alpha),             d;
         0,            0,                       0,                       1];
end

== matlab function AR4_robotv5/Subsystem12/MATLAB Function4 ==
  data: theta1 input; H output; theta2 input; theta3 input; theta4 input; theta5 input; theta6 input; X output; Y output; Z output; Rz output; Ry output; Rx output
function [H, X, Y, Z, Rz, Ry, Rx] = forward_kinematics_AR4(theta1, theta2, theta3, theta4, theta5, theta6)
% forward_kinematics_AR4 Computes the forward kinematics for the AR4 robot.
%
%   [H, X, Y, Z, Rz, Ry, Rx] = forward_kinematics_AR4(theta1, theta2, theta3, theta4, theta5, theta6)
%
%   Inputs:
%       theta1, theta2, theta3, theta4, theta5, theta6 - Joint angles (degrees)
%
%   Outputs:
%       H  - 4x4 homogeneous transformation matrix of the end-effector (mm)
%       X, Y, Z - End-effector position coordinates (mm)
%       Rz, Ry, Rx - End-effector orientation angles in degrees (ZYX Euler angles)
%
%   The AR4 robot parameters (in mm) used here are:
%       a1 = 64.2;   a2 = 305;    a3 = 0;
%       d1 = 151.27; d4 = 225.04; d6 = 37.9;
%
%   The DH parameters are defined as:
%       Joint 1: [theta1,         d1, a1, -90]
%       Joint 2: [theta2 - 90,     0,  a2,   0]
%       Joint 3: [theta3 + 180,    0,  a3,  90]
%       Joint 4: [theta4,         d4,  0,   -90]
%       Joint 5: [theta5,          0,  0,    90]
%       Joint 6: [theta6,         d6,  0,     0]

    %% Robot parameters
    a1 = 64.2;     a2 = 305;    a3 = 0;
    d1 = 151.27;   d4 = 225.04; d6 = 84.832;

    %% DH parameters
    DH1 = [theta1,       d1, a1, -90];
    DH2 = [theta2 - 90,  0,  a2,   0];
    DH3 = [theta3 + 180, 0,  a3,  90];
    DH4 = [theta4,       d4,  0,   -90];
    DH5 = [theta5,        0,  0,    90];
    DH6 = [theta6,       d6,  0,     0];

    %% Compute transformations
    A1 = computeDH(DH1);
    A2 = computeDH(DH2);
    A3 = computeDH(DH3);
    A4 = computeDH(DH4);
    A5 = computeDH(DH5);
    A6 = computeDH(DH6);

    H = A1 * A2 * A3 * A4 * A5 * A6;

    %% Extract position
    X = H(1,4);
    Y = H(2,4);
    Z = H(3,4);

    %% Extract orientation (ZYX Euler angles in degrees)
    R = H(1:3, 1:3);
    
    % Calculate Ry (pitch)
    Ry = atan2d(-R(3,1), sqrt(R(3,2)^2 + R(3,3)^2));
    
    % Check for gimbal lock (pitch near ±90°)
    if abs(abs(Ry) - 90) < eps
        % Gimbal lock case - set yaw to 0 and compute roll from alternate terms
        Rz = 0;
        Rx = atan2d(R(1,2), R(2,2));
    else
        % Normal case
        Rz = atan2d(R(2,1), R(1,1));
        Rx = atan2d(R(3,2), R(3,3));
    end
end

function A = computeDH(dh)
    theta = dh(1);
    d     = dh(2);
    a     = dh(3);
    alpha = dh(4);
    
    A = [cosd(theta), -sind(theta)*cosd(alpha),  sind(theta)*sind(alpha), a*cosd(theta);
         sind(theta),  cosd(theta)*cosd(alpha), -cosd(theta)*sind(alpha), a*sind(theta);
         0,            sind(alpha),             cosd(alpha),             d;
         0,            0,                       0,                       1];
end

== matlab function AR4_robotv5/MATLAB Function ==
  data: q input; stopFlag input
function store_joint_angles(q, stopFlag)
%#codegen

% Inputs:
%   q        : 6x1 joint angle vector
%   stopFlag : 1 if simulation is ending, 0 otherwise

persistent Q_table idx
coder.extrinsic('assignin')  % Let Simulink use this for simulation only

if isempty(Q_table)
    Q_table = zeros(10000, 6);  % Allocate storage
    idx = 1;
end

% Store current joint angles
if idx <= size(Q_table, 1)
    Q_table(idx, :) = q(:)';
    idx = idx + 1;
end

% At end of simulation, export to base workspace
if stopFlag
    assignin('base', 'JointAngleLog', Q_table(1:idx-1, :));
end

== matlab function AR4_robotv5/MATLAB Function4 ==
  data: q input; stopFlag input
function store_joint_angles(q, stopFlag)
%#codegen

% Inputs:
%   q        : 6x1 joint angle vector
%   stopFlag : 1 if simulation is ending, 0 otherwise

persistent Q_table idx
coder.extrinsic('assignin')  % Let Simulink use this for simulation only

if isempty(Q_table)
    Q_table = zeros(10000, 6);  % Allocate storage
    idx = 1;
end

% Store current joint angles
if idx <= size(Q_table, 1)
    Q_table(idx, :) = q(:)';
    idx = idx + 1;
end

% At end of simulation, export to base workspace
if stopFlag
    assignin('base', 'JointAngleLog', Q_table(1:idx-1, :));
end

== matlab function AR4_robotv5/MATLAB Function7 ==
  data: theta1 input; H output; theta2 input; theta3 input; theta4 input; theta5 input; theta6 input; q output; Rz output; Ry output; Rx output
function [H, q, Rz, Ry, Rx] = forward_kinematics_AR4(theta1, theta2, theta3, theta4, theta5, theta6)
% forward_kinematics_AR4 Computes the forward kinematics for the AR4 robot.
%
%   [H, X, Y, Z, Rz, Ry, Rx] = forward_kinematics_AR4(theta1, theta2, theta3, theta4, theta5, theta6)
%
%   Inputs:
%       theta1, theta2, theta3, theta4, theta5, theta6 - Joint angles (degrees)
%
%   Outputs:
%       H  - 4x4 homogeneous transformation matrix of the end-effector (mm)
%       X, Y, Z - End-effector position coordinates (mm)
%       Rz, Ry, Rx - End-effector orientation angles in degrees (ZYX Euler angles)
%
%   The AR4 robot parameters (in mm) used here are:
%       a1 = 64.2;   a2 = 305;    a3 = 0;
%       d1 = 151.27; d4 = 225.04; d6 = 37.9;
%
%   The DH parameters are defined as:
%       Joint 1: [theta1,         d1, a1, -90]
%       Joint 2: [theta2 - 90,     0,  a2,   0]
%       Joint 3: [theta3 + 180,    0,  a3,  90]
%       Joint 4: [theta4,         d4,  0,   -90]
%       Joint 5: [theta5,          0,  0,    90]
%       Joint 6: [theta6,         d6,  0,     0]

    %% Robot parameters
    a1 = 64.2;     a2 = 305;    a3 = 0;
    d1 = 151.27;   d4 = 225.04; d6 = 84.832;

    %% DH parameters
    DH1 = [theta1,       d1, a1, -90];
    DH2 = [theta2 - 90,  0,  a2,   0];
    DH3 = [theta3 + 180, 0,  a3,  90];
    DH4 = [theta4,       d4,  0,   -90];
    DH5 = [theta5,        0,  0,    90];
    DH6 = [theta6,       d6,  0,     0];

    %% Compute transformations
    A1 = computeDH(DH1);
    A2 = computeDH(DH2);
    A3 = computeDH(DH3);
    A4 = computeDH(DH4);
    A5 = computeDH(DH5);
    A6 = computeDH(DH6);

    H = A1 * A2 * A3 * A4 * A5 * A6;

    %% Extract position
   
        q = [H(1,4); H(2,4); H(3,4)];  % ← Cartesian position vector

    

    %% Extract orientation (ZYX Euler angles in degrees)
    R = H(1:3, 1:3);
    
    % Calculate Ry (pitch)
    Ry = atan2d(-R(3,1), sqrt(R(3,2)^2 + R(3,3)^2));
    
    % Check for gimbal lock (pitch near ±90°)
    if abs(abs(Ry) - 90) < eps
        % Gimbal lock case - set yaw to 0 and compute roll from alternate terms
        Rz = 0;
        Rx = atan2d(R(1,2), R(2,2));
    else
        % Normal case c
        Rz = atan2d(R(2,1), R(1,1));
        Rx = atan2d(R(3,2), R(3,3));
    end
end

function A = computeDH(dh)
    theta = dh(1);
    d     = dh(2);
    a     = dh(3);
    alpha = dh(4);
    
    A = [cosd(theta), -sind(theta)*cosd(alpha),  sind(theta)*sind(alpha), a*cosd(theta);
         sind(theta),  cosd(theta)*cosd(alpha), -cosd(theta)*sind(alpha), a*sind(theta);
         0,            sind(alpha),             cosd(alpha),             d;
         0,            0,                       0,                       1];
end

== matlab function AR4_robotv5/MATLAB Function8 ==
  data: theta1 input; H output; theta2 input; theta3 input; theta4 input; theta5 input; theta6 input; q output; Rz output; Ry output; Rx output
function [H, q, Rz, Ry, Rx] = forward_kinematics_AR4(theta1, theta2, theta3, theta4, theta5, theta6)
% forward_kinematics_AR4 Computes the forward kinematics for the AR4 robot.
%
%   [H, X, Y, Z, Rz, Ry, Rx] = forward_kinematics_AR4(theta1, theta2, theta3, theta4, theta5, theta6)
%
%   Inputs:
%       theta1, theta2, theta3, theta4, theta5, theta6 - Joint angles (degrees)
%
%   Outputs:
%       H  - 4x4 homogeneous transformation matrix of the end-effector (mm)
%       X, Y, Z - End-effector position coordinates (mm)
%       Rz, Ry, Rx - End-effector orientation angles in degrees (ZYX Euler angles)
%
%   The AR4 robot parameters (in mm) used here are:
%       a1 = 64.2;   a2 = 305;    a3 = 0;
%       d1 = 151.27; d4 = 225.04; d6 = 37.9;
%
%   The DH parameters are defined as:
%       Joint 1: [theta1,         d1, a1, -90]
%       Joint 2: [theta2 - 90,     0,  a2,   0]
%       Joint 3: [theta3 + 180,    0,  a3,  90]
%       Joint 4: [theta4,         d4,  0,   -90]
%       Joint 5: [theta5,          0,  0,    90]
%       Joint 6: [theta6,         d6,  0,     0]

    %% Robot parameters
    a1 = 64.2;     a2 = 305;    a3 = 0;
    d1 = 151.27;   d4 = 225.04; d6 = 84.832;

    %% DH parameters
    DH1 = [theta1,       d1, a1, -90];
    DH2 = [theta2 - 90,  0,  a2,   0];
    DH3 = [theta3 + 180, 0,  a3,  90];
    DH4 = [theta4,       d4,  0,   -90];
    DH5 = [theta5,        0,  0,    90];
    DH6 = [theta6,       d6,  0,     0];

    %% Compute transformations
    A1 = computeDH(DH1);
    A2 = computeDH(DH2);
    A3 = computeDH(DH3);
    A4 = computeDH(DH4);
    A5 = computeDH(DH5);
    A6 = computeDH(DH6);

    H = A1 * A2 * A3 * A4 * A5 * A6;

    %% Extract position
   
        q = [H(1,4); H(2,4); H(3,4)];  % ← Cartesian position vector

    

    %% Extract orientation (ZYX Euler angles in degrees)
    R = H(1:3, 1:3);
    
    % Calculate Ry (pitch)
    Ry = atan2d(-R(3,1), sqrt(R(3,2)^2 + R(3,3)^2));
    
    % Check for gimbal lock (pitch near ±90°)
    if abs(abs(Ry) - 90) < eps
        % Gimbal lock case - set yaw to 0 and compute roll from alternate terms
        Rz = 0;
        Rx = atan2d(R(1,2), R(2,2));
    else
        % Normal case c
        Rz = atan2d(R(2,1), R(1,1));
        Rx = atan2d(R(3,2), R(3,3));
    end
end

function A = computeDH(dh)
    theta = dh(1);
    d     = dh(2);
    a     = dh(3);
    alpha = dh(4);
    
    A = [cosd(theta), -sind(theta)*cosd(alpha),  sind(theta)*sind(alpha), a*cosd(theta);
         sind(theta),  cosd(theta)*cosd(alpha), -cosd(theta)*sind(alpha), a*sind(theta);
         0,            sind(alpha),             cosd(alpha),             d;
         0,            0,                       0,                       1];
end

== matlab function AR4_robotv5/MATLAB Function9 ==
  data: theta1 input; H output; theta2 input; theta3 input; theta4 input; theta5 input; theta6 input; q output; Rz output; Ry output; Rx output
function [H, q, Rz, Ry, Rx] = forward_kinematics_AR4(theta1, theta2, theta3, theta4, theta5, theta6)
% forward_kinematics_AR4 Computes the forward kinematics for the AR4 robot.
%
%   [H, X, Y, Z, Rz, Ry, Rx] = forward_kinematics_AR4(theta1, theta2, theta3, theta4, theta5, theta6)
%
%   Inputs:
%       theta1, theta2, theta3, theta4, theta5, theta6 - Joint angles (degrees)
%
%   Outputs:
%       H  - 4x4 homogeneous transformation matrix of the end-effector (mm)
%       X, Y, Z - End-effector position coordinates (mm)
%       Rz, Ry, Rx - End-effector orientation angles in degrees (ZYX Euler angles)
%
%   The AR4 robot parameters (in mm) used here are:
%       a1 = 64.2;   a2 = 305;    a3 = 0;
%       d1 = 151.27; d4 = 225.04; d6 = 37.9;
%
%   The DH parameters are defined as:
%       Joint 1: [theta1,         d1, a1, -90]
%       Joint 2: [theta2 - 90,     0,  a2,   0]
%       Joint 3: [theta3 + 180,    0,  a3,  90]
%       Joint 4: [theta4,         d4,  0,   -90]
%       Joint 5: [theta5,          0,  0,    90]
%       Joint 6: [theta6,         d6,  0,     0]

    %% Robot parameters
    a1 = 64.2;     a2 = 305;    a3 = 0;
    d1 = 151.27;   d4 = 225.04; d6 = 84.832;

    %% DH parameters
    DH1 = [theta1,       d1, a1, -90];
    DH2 = [theta2 ,  0,  a2,   0];
    DH3 = [theta3 , 0,  a3,  90];
    DH4 = [theta4,       d4,  0,   -90];
    DH5 = [theta5,        0,  0,    90];
    DH6 = [theta6,       d6,  0,     0];

    %% Compute transformations
    A1 = computeDH(DH1);
    A2 = computeDH(DH2);
    A3 = computeDH(DH3);
    A4 = computeDH(DH4);
    A5 = computeDH(DH5);
    A6 = computeDH(DH6);

    H = A1 * A2 * A3 * A4 * A5 * A6;

    %% Extract position
   
        q = [H(1,4); H(2,4); H(3,4)];  % ← Cartesian position vector

    

    %% Extract orientation (ZYX Euler angles in degrees)
    R = H(1:3, 1:3);
    
    % Calculate Ry (pitch)
    Ry = atan2d(-R(3,1), sqrt(R(3,2)^2 + R(3,3)^2));
    
    % Check for gimbal lock (pitch near ±90°)
    if abs(abs(Ry) - 90) < eps
        % Gimbal lock case - set yaw to 0 and compute roll from alternate terms
        Rz = 0;
        Rx = atan2d(R(1,2), R(2,2));
    else
        % Normal case c
        Rz = atan2d(R(2,1), R(1,1));
        Rx = atan2d(R(3,2), R(3,3));
    end
end

function A = computeDH(dh)
    theta = dh(1);
    d     = dh(2);
    a     = dh(3);
    alpha = dh(4);
    
    A = [cosd(theta), -sind(theta)*cosd(alpha),  sind(theta)*sind(alpha), a*cosd(theta);
         sind(theta),  cosd(theta)*cosd(alpha), -cosd(theta)*sind(alpha), a*sind(theta);
         0,            sind(alpha),             cosd(alpha),             d;
         0,            0,                       0,                       1];
end

== matlab function AR4_robotv5/MATLAB Function10 ==
  data: theta1 input; H output; theta2 input; theta3 input; theta4 input; theta5 input; theta6 input; q output; Rz output; Ry output; Rx output
function [H, q, Rz, Ry, Rx] = forward_kinematics_AR4(theta1, theta2, theta3, theta4, theta5, theta6)
% forward_kinematics_AR4 Computes the forward kinematics for the AR4 robot.
%
%   [H, X, Y, Z, Rz, Ry, Rx] = forward_kinematics_AR4(theta1, theta2, theta3, theta4, theta5, theta6)
%
%   Inputs:
%       theta1, theta2, theta3, theta4, theta5, theta6 - Joint angles (degrees)
%
%   Outputs:
%       H  - 4x4 homogeneous transformation matrix of the end-effector (mm)
%       X, Y, Z - End-effector position coordinates (mm)
%       Rz, Ry, Rx - End-effector orientation angles in degrees (ZYX Euler angles)
%
%   The AR4 robot parameters (in mm) used here are:
%       a1 = 64.2;   a2 = 305;    a3 = 0;
%       d1 = 151.27; d4 = 225.04; d6 = 37.9;
%
%   The DH parameters are defined as:
%       Joint 1: [theta1,         d1, a1, -90]
%       Joint 2: [theta2 - 90,     0,  a2,   0]
%       Joint 3: [theta3 + 180,    0,  a3,  90]
%       Joint 4: [theta4,         d4,  0,   -90]
%       Joint 5: [theta5,          0,  0,    90]
%       Joint 6: [theta6,         d6,  0,     0]

    %% Robot parameters
    a1 = 64.2;     a2 = 305;    a3 = 0;
    d1 = 151.27;   d4 = 225.04; d6 = 84.832;

    %% DH parameters
    DH1 = [theta1,       d1, a1, -90];
    DH2 = [theta2 - 90,  0,  a2,   0];
    DH3 = [theta3 + 180, 0,  a3,  90];
    DH4 = [theta4,       d4,  0,   -90];
    DH5 = [theta5,        0,  0,    90];
    DH6 = [theta6,       d6,  0,     0];

    %% Compute transformations
    A1 = computeDH(DH1);
    A2 = computeDH(DH2);
    A3 = computeDH(DH3);
    A4 = computeDH(DH4);
    A5 = computeDH(DH5);
    A6 = computeDH(DH6);

    H = A1 * A2 * A3 * A4 * A5 * A6;

    %% Extract position
   
        q = [H(1,4); H(2,4); H(3,4)];  % ← Cartesian position vector

    

    %% Extract orientation (ZYX Euler angles in degrees)
    R = H(1:3, 1:3);
    
    % Calculate Ry (pitch)
    Ry = atan2d(-R(3,1), sqrt(R(3,2)^2 + R(3,3)^2));
    
    % Check for gimbal lock (pitch near ±90°)
    if abs(abs(Ry) - 90) < eps
        % Gimbal lock case - set yaw to 0 and compute roll from alternate terms
        Rz = 0;
        Rx = atan2d(R(1,2), R(2,2));
    else
        % Normal case c
        Rz = atan2d(R(2,1), R(1,1));
        Rx = atan2d(R(3,2), R(3,3));
    end
end

function A = computeDH(dh)
    theta = dh(1);
    d     = dh(2);
    a     = dh(3);
    alpha = dh(4);
    
    A = [cosd(theta), -sind(theta)*cosd(alpha),  sind(theta)*sind(alpha), a*cosd(theta);
         sind(theta),  cosd(theta)*cosd(alpha), -cosd(theta)*sind(alpha), a*sind(theta);
         0,            sind(alpha),             cosd(alpha),             d;
         0,            0,                       0,                       1];
end

== matlab function AR4_robotv5/MATLAB Function12 ==
  data: q input; stopFlag input
function store_joint1_angle(q, stopFlag)
%#codegen

persistent Q_table idx
coder.extrinsic('assignin')

if isempty(Q_table)
    Q_table = zeros(10000, 1);  % for 1 joint only
    idx = 1;
end

% Store current joint angle
if idx <= size(Q_table, 1)
    Q_table(idx) = q;
    idx = idx + 1;
end

% On simulation end, remove trailing repeated values and export
if stopFlag
    data = Q_table(1:idx-1);

    % Remove repeated identical values at the end
    last_val = data(end);
    i = length(data);
    while i > 1 && data(i-1) == last_val
        i = i - 1;
    end
    compressed_data = data(1:i);  % Keep only one instance of trailing repeats

    assignin('base', 'Joint1AngleLog', compressed_data);
end

== matlab function AR4_robotv5/MATLAB Function13 ==
  data: q input; stopFlag input
function store_position(q, stopFlag)
%#codegen

% Inputs:
%   q        : 3x1 position vector [x; y; z]
%   stopFlag : 1 if simulation is ending, 0 otherwise

persistent Q_table idx
coder.extrinsic('assignin')  % Needed to export to MATLAB base workspace

if isempty(Q_table)
    Q_table = zeros(10000, 3);  % Preallocate for up to 10,000 steps
    idx = 1;
end

% Store the current position
if idx <= size(Q_table, 1)
    Q_table(idx, :) = q(:)';  % Store as a row
    idx = idx + 1;
end

% Export to base workspace at the end of simulation
if stopFlag
    assignin('base', 'PositionLog', Q_table(1:idx-1, :));
end

== matlab function AR4_robotv5/MATLAB Function14 ==
  data: q input; stopFlag input
function store_joint_angles(q, stopFlag)
%#codegen

% Inputs:
%   q        : 6x1 joint angle vector
%   stopFlag : 1 if simulation is ending, 0 otherwise

persistent Q_table idx
coder.extrinsic('assignin')  % Let Simulink use this for simulation only

if isempty(Q_table)
    Q_table = zeros(10000, 6);  % Allocate storage
    idx = 1;
end

% Store current joint angles
if idx <= size(Q_table, 1)
    Q_table(idx, :) = q(:)';
    idx = idx + 1;
end

% At end of simulation, export to base workspace
if stopFlag
    assignin('base', 'JointAngleLog', Q_table(1:idx-1, :));
end

== matlab function AR4_robotv5/MATLAB Function15 ==
  data: q input; stopFlag input
function store_joint_angles(q, stopFlag)
%#codegen

% Inputs:
%   q        : 6x1 joint angle vector
%   stopFlag : 1 if simulation is ending, 0 otherwise

persistent Q_table idx
coder.extrinsic('assignin')  % Let Simulink use this for simulation only

if isempty(Q_table)
    Q_table = zeros(10000, 6);  % Allocate storage
    idx = 1;
end

% Store current joint angles
if idx <= size(Q_table, 1)
    Q_table(idx, :) = q(:)';
    idx = idx + 1;
end

% At end of simulation, export to base workspace
if stopFlag
    assignin('base', 'JointAngleLog', Q_table(1:idx-1, :));
end

== matlab function AR4_robotv5/MATLAB Function16 ==
  data: joint1_angles input; q output; time_now input
function q = generate_bspline_point(joint1_angles, time_now)
%#codegen
% Inputs:
%   joint1_angles : [1 x N] control points
%   time_now      : scalar time input (e.g., from clock block)
% Output:
%   q             : interpolated joint value at time_now

% Ensure row vector for bsplinepolytraj
controlPoints = joint1_angles(:)';  % 1xN

% Time interval
timeInterval = [0 7];  % adjust as needed

% Evaluate only at the current time
[q_out, ~, ~] = bsplinepolytraj(controlPoints, timeInterval, time_now);

% Output as scalar for plotting to Scope
q = q_out;
end

== matlab function AR4_robotv5/MATLAB Function17 ==
  data: joint1_angles input; q output; time_now input
function q = generate_quintic_bspline_point(joint1_angles, time_now)
%#codegen

coder.extrinsic('spapi', 'fnval', 'linspace', 'length');

% Predefine output type for Simulink compatibility
q = 0;  % scalar double (required for codegen to know output shape)

% Force row vector input
controlPoints = joint1_angles(:)';

% Define knot (time) vector matching the control points
n = length(controlPoints);
t_waypoints = linspace(0, 7, n);  % time for waypoints

% Create the spline and evaluate it (only works in simulation)
pp = spapi(6, t_waypoints, controlPoints);   % order 6 → quintic
q = fnval(pp, time_now);                     % evaluate at this time
